simulink model "Use_the_phase_locked_loop_block_to_extract"  (R2021a)
settings: Solver=VariableStepAuto  StartTime=0.0  StopTime=10.0  RelTol=1e-3
libraries: commsynccomp2 x1, simulink x1
settings Model: Creator=Fatiha  LastModifiedBy=Fatiha

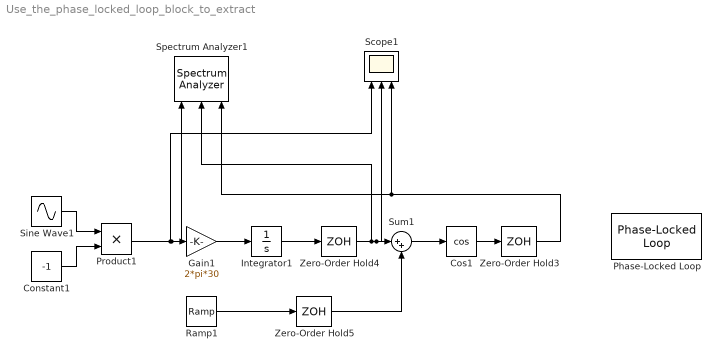
== system Use_the_phase_locked_loop_block_to_extract ==
  Constant1 : Constant  Value=-1  SampleTime=0.0001
  Cos1 : Trigonometry  Operator=cos  OutputSignalType=real
  Gain1 : Gain  Gain=2*pi*30
  Integrator1 : Integrator
  Phase-Locked Loop : commsynccomp2/Phase-Locked Loop  Fn="[3.0002  0  40002]"  Fd="[1   67.46   2270.9   40002]"  Kvco=1  Fc=100  Ph=0  Ac=1
      settings: SourceProductBaseCode=CM
  Product1 : Product
  Ramp1 : simulink/Sources/Ramp  slope=2*pi*200  start=0  InitialOutput=0
  Scope1 : Scope  NumInputPorts=3
  Sine Wave1 : Sin  Frequency=2*pi*50  SampleTime=0.00001
  Spectrum Analyzer1 : SpectrumAnalyzer  NumInputPorts=3
  Sum1 : Sum  Inputs=|++
  Zero-Order Hold3 : ZeroOrderHold  SampleTime=0.00001
  Zero-Order Hold4 : ZeroOrderHold  SampleTime=0.00001
  Zero-Order Hold5 : ZeroOrderHold  SampleTime=0.00001
  wires:
  Zero-Order Hold4/1 -> Scope1/2, Sum1/1, Spectrum Analyzer1/2
  Integrator1/1 -> Zero-Order Hold4/1
  Ramp1/1 -> Zero-Order Hold5/1
  Product1/1 -> Scope1/1, Spectrum Analyzer1/1, Gain1/1
  Gain1/1 -> Integrator1/1
  Cos1/1 -> Zero-Order Hold3/1
  Zero-Order Hold5/1 -> Sum1/2
  Sine Wave1/1 -> Product1/1
  Sum1/1 -> Cos1/1
  Constant1/1 -> Product1/2
  Zero-Order Hold3/1 -> Scope1/3, Spectrum Analyzer1/3
